simulink model "Bruening_4t_showshuffle"  (R2015a)
settings: Solver=ode4  SolverMode=MultiTasking  StartTime=0.0  StopTime=inf  FixedStep=BKIN_STEP_TIME  RelTol=1e-3
StartFcn:
  |  warndlg('Dexterit-E models cannot run under simulation. Please compile your model and run it from within Dexterit-E.');set_param(bdroot,'SimulationCommand','stop')
model workspace (MAT data in the model file):
  BKIN_STEP_TIME = 0.00025
  col_x = 1
  col_y = 2
  E_TARGET_ON = 3
  E_HOLD_AT_TARGET = 5
  LOGICAL_RADIUS = 4
  START_TARGET_COL = 1
  END_TARGET_COL = 2
  ROTATION_CENTER = 5
  WAIT_AT_1stTARGET_COL = 7
  MAXREACHTIME_COL = 8
  DELAY_POSTTRIAL_COL = 9
  E_STAY_CENTER = 2
  VISUAL_RADIUS = 3
  COLOR = 5
  ALTCOLOR = 6
  STROKECOLOUR = 7
  STROKEWIDTH = 9
  TARGET_EGG = 6
  LABEL_TEXT = 12
  LABEL_COLOUR = 13
  LABEL_HEIGHT = 14
  TEXT_DISPLAY_TARGET = 10
  ALTSTROKECOLOUR = 8
  SEGMENT_COUNT = 11
  E_TARGET_MISS = 6
  END_X = 10
  END_Y = 11
  E_LEFT_RING = 4
  E_START_BLOCK = 10
  BKIN_KINEMATIC_FRAME_SIZE = 400
  E_NO_EVENT = 1
  TARGET_IN_USE = 3
  R_PROB = 4
  E_R_TARG1 = 7
  E_M_TARG1 = 12
  E_R_TARG2 = 8
  E_M_TARG2 = 13
  E_R_TARG3 = 9
  E_M_TARG3 = 14
  E_R_TARG4 = 11
  E_M_TARG4 = 15
  WAIT_TIME = 12
  TONE_DURATION = 13
  FLASH_INTER = 14
  FLASH_NUM = 15
  BREAK_T1 = 16
  BREAK_T2 = 17
  ALTVISUAL_RADIUS = 15
  ALTCOLOR2 = 16
undefined symbols (not defined in the file or in its folder): slselsubs
libraries: Video x15, simulink x12, xpcrtudplib x12, xpcutilitieslib x10, xpcobsoletelib x8, ethercat x2, General x2, slrtlib x2, KINARM_general x1
(part 5 of 6)

== matlab function Bruening_4t_showshuffle/DataLogging/Poll KINARM/PMAC Subsystem/read_pmac/Robot_data_builder ==
  data: bR1HasSecondardy input; bR2HasSecondardy input; robot1Data input; robot2Data input; robot1PrimaryEncData input; robot2PrimaryEncData input; robot1DataOut output; robot2DataOut output; servoCounter input; plccVer input; robot1PrimaryEncDataOut output; robot2PrimaryEncDataOut output
function [robot1DataOut, robot2DataOut, robot1PrimaryEncDataOut, robot2PrimaryEncDataOut] = convertPMACValues(bR1HasSecondardy, bR2HasSecondardy, robot1Data, robot2Data, robot1PrimaryEncData, robot2PrimaryEncData, servoCounter, plccVer)

    persistent robot1Struct robot2Struct robot1StructPrimary robot2StructPrimary servoValuesR1 servoValuesR2
    
    if isempty(robot1Struct)
        robot1Struct = getStruct();
        robot2Struct = getStruct();
        robot1StructPrimary = getStruct();
        robot2StructPrimary = getStruct();
        servoValuesR1 = zeros(5, 1);
        servoValuesR2 = zeros(5, 1);
    end
    
    if plccVer < 7
        robot1DataOut = robot1Data;
        robot2DataOut = robot2Data;
        robot1PrimaryEncDataOut = robot1PrimaryEncData;
        robot2PrimaryEncDataOut = robot2PrimaryEncData;
        return
    end
    
    if servoCounter(1) ~= servoValuesR1(1)
        robot1Struct = updatePositions(robot1Struct, robot1Data, bR1HasSecondardy);
        robot1StructPrimary = updatePositions(robot1StructPrimary, robot1PrimaryEncData, 0);
        servoValuesR1 = insertVal(servoValuesR1, servoCounter(1));
        robot1Struct = calculateVelAcc(robot1Struct, servoValuesR1, robot1Data);
        robot1StructPrimary = calculateVelAcc(robot1StructPrimary, servoValuesR1, robot1PrimaryEncData);
    end
    
    if servoCounter(2) ~= servoValuesR2(1)
        robot2Struct = updatePositions(robot2Struct, robot2Data, bR2HasSecondardy);
        robot2StructPrimary = updatePositions(robot2StructPrimary, robot2PrimaryEncData, 0);
        servoValuesR2 = insertVal(servoValuesR2, servoCounter(2));
        robot2Struct = calculateVelAcc(robot2Struct, servoValuesR2, robot2Data);
        robot2StructPrimary = calculateVelAcc(robot2StructPrimary, servoValuesR2, robot2PrimaryEncData);
    end
    
    robot1DataOut = insertVelAcc(robot1Data, robot1Struct);
    robot2DataOut = insertVelAcc(robot2Data, robot2Struct);

    robot1PrimaryEncDataOut = insertVelAcc(robot1PrimaryEncData, robot1StructPrimary);
    robot2PrimaryEncDataOut = insertVelAcc(robot2PrimaryEncData, robot2StructPrimary);
    
    %We used to provide a filtered velocity, but we can't with EtherCAT and
    %it was not being used anywhere anyway. 
    robot1DataOut(7:8) = robot1DataOut(3:4);
    robot2DataOut(7:8) = robot2DataOut(3:4);
end


function robotDataOut = insertVelAcc(robotData, robotStruct)
    robotDataOut = robotData(:);
    robotDataOut(3) = robotStruct.shoVel(1);
    robotDataOut(4) = robotStruct.elbVel(1);
    robotDataOut(5) = robotStruct.shoAcc;
    robotDataOut(6) = robotStruct.elbAcc;
end

function st=getStruct()
    st = struct('shoPos', zeros(5, 1), 'elbPos', zeros(5, 1), ...
        'shoVel', zeros(5, 1), 'elbVel', zeros(5, 1), ...
        'shoAcc', 0, 'elbAcc', 0, 'bHasSecondary', 0);
end

function robotStruct = updatePositions(robotStruct, robotData, bHasSecondardy)
    robotStruct.shoPos = insertVal(robotStruct.shoPos, robotData(1));
    robotStruct.elbPos = insertVal(robotStruct.elbPos, robotData(2));
    robotStruct.bHasSecondary = bHasSecondardy;
end

function arr=insertVal(arr, v)
    arr = circshift(arr, 1);
    arr(1) = v;
end

function robotStructOut=calculateVelAcc(robotStruct, servoValues, robotData)
    %matches from PMAC code
    robotStructOut = robotStruct;
    servoTimeStep = (7427414.0/8388608.0) / 1000; 
    %do not name this anything that will make it the first variable name in
    %this method alphabetically. Seriously. With the name "duration" compiling
    %a model would work in 2010a, but nothing higher. Most models would compile,
    %but the verification task would not!
    stepDuration = 0;
    
    if robotStruct.bHasSecondary
        stepDuration = ((servoValues(1) - servoValues(2)) * servoTimeStep);
        if stepDuration == 0
            shoVel = robotStruct.shoVel(1);
            elbVel = robotStruct.elbVel(1);
        else
            shoVel = (robotStruct.shoPos(1) - robotStruct.shoPos(2)) / stepDuration;
            elbVel = (robotStruct.elbPos(1) - robotStruct.elbPos(2)) / stepDuration;        
        end
    else
        shoVel = robotData(3);
        elbVel = robotData(4);
    end
    
    robotStructOut.shoVel = insertVal(robotStruct.shoVel, shoVel);
    robotStructOut.elbVel = insertVal(robotStruct.elbVel, elbVel);

    if robotStruct.bHasSecondary        
        if stepDuration == 0
            shoAcc = robotStruct.shoAcc;
            elbAcc = robotStruct.elbAcc;
        else
            shoAcc = (robotStruct.shoVel(1) - robotStruct.shoVel(2)) / stepDuration;
            elbAcc = (robotStruct.elbVel(1) - robotStruct.elbVel(2)) / stepDuration;        
        end
    else
        stepDuration = ((servoValues(1) - servoValues(5)) * servoTimeStep);
        shoAcc = (robotStruct.shoVel(1) - robotStruct.shoVel(5)) / stepDuration;
        elbAcc = (robotStruct.elbVel(1) - robotStruct.elbVel(5)) / stepDuration;        
    end    
    
    robotStructOut.shoAcc = shoAcc;
    robotStructOut.elbAcc = elbAcc;
end

== matlab function Bruening_4t_showshuffle/DataLogging/Poll KINARM/PMAC Subsystem/read_pmac/filter_velocities ==
  data: robot1Data input; robot2Data input; robot1DataOut output; robot2DataOut output; servoCounters input; plccVer input
function [robot1DataOut, robot2DataOut] = filterVelocities(robot1Data, robot2Data, servoCounters, plccVer)

    persistent robot1Struct robot2Struct
    POLES = 2;
    
    if isempty(robot1Struct)
        robot1Struct = getStruct(POLES);
        robot2Struct = getStruct(POLES);
    end
    
    if plccVer < 7
        robot1DataOut = robot1Data;
        robot2DataOut = robot2Data;
        return
    end
    
    robot1DataOut = robot1Data(:);
    robot2DataOut = robot2Data(:);
    
    robot1Struct = updateValues(robot1Struct, robot1Data, servoCounters(1), POLES);
    robot2Struct = updateValues(robot2Struct, robot2Data, servoCounters(2), POLES);
        
    %We used to provide a filtered velocity, but we can't with EtherCAT and
    %it was not being used anywhere anyway. 
    robot1DataOut(7:8) = [robot1Struct.shoVelFilt(POLES + 1), robot1Struct.elbVelFilt(POLES + 1)];
    robot2DataOut(7:8) = [robot2Struct.shoVelFilt(POLES + 1), robot2Struct.elbVelFilt(POLES + 1)];
end


function st=getStruct(poles)
    valueCount = poles + 1;
    st = struct('shoVel', zeros(valueCount, 1), 'elbVel', zeros(valueCount, 1), ...
        'shoVelFilt', zeros(valueCount, 1), 'elbVelFilt', zeros(valueCount, 1), ...
        'servoCounter', zeros(valueCount, 1));
end

function arr=insertVal(arr, v)
    arr = circshift(arr, -1);
    arr(length(arr)) = v;
end

function robotStruct = updateValues(robotStruct, robotData, servoCounter, POLES)
    if servoCounter == robotStruct.servoCounter(POLES + 1)
        return
    end
    
    robotStruct.servoCounter = insertVal(robotStruct.servoCounter, servoCounter);
    
    [robotStruct.shoVel, robotStruct.shoVelFilt] = filterJoint(robotStruct.shoVel, robotStruct.shoVelFilt, robotData(3), POLES);
    [robotStruct.elbVel, robotStruct.elbVelFilt] = filterJoint(robotStruct.elbVel, robotStruct.elbVelFilt, robotData(4), POLES);
end

function [velocitiesOut, velFilt] = filterJoint(velocities, filtVelocities, newVelocity, POLES)

%all filter constants from http://www-users.cs.york.ac.uk/~fisher/cgi-bin/mkfscript

    %GAIN = 4.143204922e+03; % 1KHz gain
    GAIN = 1.342624471e+03; %1.129 KHz gain (PMAC speed)
    
    %FILTER_VALUES = [-0.9565436765, 1.9555782403]; % 1KHz
    FILTER_VALUES = [-0.9243128082, 1.9213335686]; % 1.129 KHz
    
    velocitiesOut = insertVal(velocities, newVelocity / GAIN);
    velFilt = insertVal(filtVelocities, 0);

    velFilt(POLES + 1) = velocitiesOut(1) + ...
         velocitiesOut(2) * 2.0 + ...
         velocitiesOut(3) + ...
         velFilt(1) * FILTER_VALUES(1) + ...
         velFilt(2) * FILTER_VALUES(2);
    
     if isnan(velFilt(POLES + 1)) || isinf(velFilt(POLES + 1))
         velFilt(POLES + 1) = 0;
    end
end

== matlab function Bruening_4t_showshuffle/DataLogging/Poll KINARM/PMAC Subsystem/update settings/update status format ==
  data: pmacStatus input; outStatus output
function outStatus = fcn(pmacStatus)
%#eml

outStatus = zeros(1, 7, 'uint32');
outStatus(5:6) = pmacStatus(2:3);

STATUS_FUNCTIONING = uint32(0);
STATUS_READY = uint32(1);
STATUS_FAULTED = uint32(2);

%Each motor has 2 possible states: 0 working, 1 faulted. The READY state is only used by EtherCAT
for n=0:3
    motor = bitand( bitshift(pmacStatus(1), -n), 1);
    if motor == 1
       outStatus(n + 1) =  STATUS_FAULTED;
    else
        outStatus(n + 1) = STATUS_FUNCTIONING;
    end
end

== matlab function Bruening_4t_showshuffle/DataLogging/Poll KINARM/constants/arm1/decode robot ==
  data: system_type input; robot_type input; isEP output; robot_version input; isHumanEXO output; isNHPEXO output; isClassicExo output; isUTSEXO output; isPMAC output; isECAT output
function [isEP, isHumanEXO, isNHPEXO, isClassicExo, isUTSEXO, isPMAC, isECAT] = fcn(system_type, robot_type, robot_version)
%#eml
isEP = 0;
isHumanEXO = 0;
isNHPEXO = 0;
isClassicExo = 0;
isUTSEXO = 0;
isPMAC = 0;
isECAT = 0;

if robot_type == 0
    isHumanEXO = 1;    
    if robot_version == 1
        isClassicExo = 1;        
    elseif robot_version == 2
        isUTSEXO = 1;
    end    
elseif robot_type == 1
    isEP = 1;
elseif robot_type == 2
    isNHPEXO = 1;        
    if robot_version == 1
        isClassicExo = 1;        
    elseif robot_version == 2
        isUTSEXO = 1;
    end
end

if system_type == 1
   isPMAC = 1;
elseif system_type == 2
    isECAT = 1;
end

== matlab function Bruening_4t_showshuffle/DataLogging/Poll KINARM/constants/arm2/decode robot ==
  data: system_type input; robot_type input; isEP output; robot_version input; isHumanEXO output; isNHPEXO output; isClassicExo output; isUTSEXO output; isPMAC output; isECAT output
function [isEP, isHumanEXO, isNHPEXO, isClassicExo, isUTSEXO, isPMAC, isECAT] = fcn(system_type, robot_type, robot_version)
%#eml
isEP = 0;
isHumanEXO = 0;
isNHPEXO = 0;
isClassicExo = 0;
isUTSEXO = 0;
isPMAC = 0;
isECAT = 0;

if robot_type == 0
    isHumanEXO = 1;    
    if robot_version == 1
        isClassicExo = 1;        
    elseif robot_version == 2
        isUTSEXO = 1;
    end    
elseif robot_type == 1
    isEP = 1;
elseif robot_type == 2
    isNHPEXO = 1;        
    if robot_version == 1
        isClassicExo = 1;        
    elseif robot_version == 2
        isUTSEXO = 1;
    end
end

if system_type == 1
   isPMAC = 1;
elseif system_type == 2
    isECAT = 1;
end

== matlab function Bruening_4t_showshuffle/DataLogging/Poll Force Plates/plate2/parse packet 1 ==
  data: packet input; forces output; moments output; timer output; calibration input; gain input; ain_slope input; ain_offset input; orientation input; zero_voltage input
function [forces, moments, timer] = fcn(packet, calibration, gain, ain_slope, ain_offset, orientation, zero_voltage)
    %This pulls voltages and timer infomation from the packet we got back from
    %the lab jack.
    
    voltages = zeros(1, 8);
    timers = zeros(1, 3);

    for n = 1:8
        bits = readUShort(packet, 13 + ((n - 1)*2));
        voltages(n) = binaryToCalibratedAnalogVoltage(bits, ain_slope, ain_offset);
    end
    
    for n = 1:3
        timers(n) = readUInt(packet, 53 + ((n - 1)*4));
    end
    
    %convert the time stamp to a time in seconds.
    timer = timers(1) / 750000.0; 
    
    %all voltages are between -2.5 to 2.5, here we are normalizeing what we read to zero.
    voltages = voltages - zero_voltage;
    voltages = voltages(1:8); % only the first 8 channels matter.
    
    %using the calibration matrix we convert the to the forces and moments
    values = calibration * (voltages / gain)';
    forces = values(1:3);
    moments = values(4:6);
    
	%reverse the Z force to get it into global coordinates.
	forces(3) = -forces(3);

	%considering the positions of the cables push all measures into global coordinates
    if orientation == 0
        forces(2) = -forces(2);
        moments(2) = -moments(2);
    elseif orientation == 90
        y = forces(2);
        forces(2) = -forces(1);
        forces(1) = -y;

        y = moments(2);
        moments(2) = -moments(1);
        moments(1) = -y;
	elseif orientation == 180
        forces(1) = -forces(1);        
        moments(1) = -moments(1);        
    elseif orientation == 270
        y = forces(2);
        forces(2) = forces(1);
        forces(1) = y;

		y = moments(2);
        moments(2) = moments(1);
        moments(1) = y;
    end
end

function val = readUShort(data, offset)
    p1 = uint32(data(offset));
    p2 = uint32(data(offset + 1));
    val = double(p1 + (p2 * 256));
end

function val = readUInt(data, offset)
    p1 = uint32(data(offset));
    p2 = uint32(data(offset + 1));
    p3 = uint32(data(offset + 2));
    p4 = uint32(data(offset + 3));
    val = double(p1 + (p2 * 256) + (p3 * 2^16) + (p4 * 2^24));
end

function voltage = binaryToCalibratedAnalogVoltage(bits, ain_slope, ain_offset)
    voltage = (bits * ain_slope) + ain_offset;
end

== matlab function Bruening_4t_showshuffle/DataLogging/Poll KINARM/createKINData/Create KINARM Data Array ==
  data: robot_calibrations input; robot_hardware_settings input; force_sensor_data input; robot_data input; servo_update_count input; delay_estimates input; primary_encoder_data input; ep_calibration_button_bitfield input; torque_command input; hand_feedback_settings input; kinarm_data output; dominant_arm input; primary_encoder_data_out output; gaze_data input
% This function constructs a matrix of KINARM-related data called "KINdata". This matrix consists of three rows: the first two are each
% for data related to the respective robot (i.e. row 1 is for robot 1 data, row 2 for robot 2 data, etc.), and the third row is for data
% not specific to either arm. Each row of the matrix is currently of length 50, though not all elements in each row are used.
function [kinarm_data, primary_encoder_data_out]= create_KINARM_data_array(robot_calibrations, robot_hardware_settings, force_sensor_data, ...
                                                      robot_data, servo_update_count, delay_estimates, primary_encoder_data, ...
                                                      ep_calibration_button_bitfield, torque_command, hand_feedback_settings, dominant_arm, gaze_data)

kinarm_data = zeros(3,50);
primary_encoder_data_out = zeros(2,6);

% Create the rows of robot-specific data. The utility function create_robot_row is used to assemble the values for each row. 
% The last section of that function (in which the row elements are assigned individually) documents the row contents.
kinarm_data(1,:) = create_robot_row(robot_calibrations(1:8), robot_hardware_settings(1:12), ...
                                    force_sensor_data(1:7), robot_data(1:10), torque_command(1:2));

kinarm_data(2,:) = create_robot_row(robot_calibrations(9:16), robot_hardware_settings(13:24), ...
                                    force_sensor_data(8:14), robot_data(11:20), torque_command(3:4));
								
% Create the last row of KINdata, which contains information not specific to any single arm.
kinarm_data(3,1) = dominant_arm;                     % dominant KINARM for the experiment (1: arm 1, 2: arm 2)
kinarm_data(3,2) = hand_feedback_settings(5);        % duration of feed forward for position of hand feedback (s)
kinarm_data(3,3) = hand_feedback_settings(1);        % hand feedback arm (0: none, 1: dominant, 2: non-dominant, 3: both, 4: controlled by task program)
kinarm_data(3,4) = hand_feedback_settings(2);        % hand feedback settings source (0: GUI, 1: from task program)
kinarm_data(3,5) = hand_feedback_settings(4);        % feedback colour (RRRGGGBBB string converted to integer)
kinarm_data(3,6) = hand_feedback_settings(3);        % feedback radius (m)
kinarm_data(3,7) = 1;                                % global load enable set by BKIN client software (no longer an option; thus always on)
kinarm_data(3,8) = delay_estimates(1);               % primary encoders velocity delay estimate (s)
kinarm_data(3,9) = delay_estimates(2);               % primary encoders acceleration delay estimate (s)
kinarm_data(3,10) = delay_estimates(3);              % secondary encoders velocity delay estimate (s)
kinarm_data(3,11) = delay_estimates(4);              % secondary encoders acceleration delay estimate (s)
kinarm_data(3,12) = servo_update_count;              % servo update count
kinarm_data(3,13) = ep_calibration_button_bitfield;  % EP calibration button status bitfield

gaze_available = gaze_data(1);
kinarm_data(3,14) = gaze_available;              % is Gaze tracking hardware available
kinarm_data(3,15) = hand_feedback_settings(6);   % Gaze feedback (0: on, 1: controlled by task program)

if gaze_available
    kinarm_data(3,16) = gaze_data(2);            % Gaze X location in global coordinates
    kinarm_data(3,17) = gaze_data(3);            % Gaze Y location in global coordinates
    kinarm_data(3,18) = gaze_data(4);            % Gaze Timestamp in seconds
    kinarm_data(3,19) = gaze_data(5);            % Gaze pupil area
    kinarm_data(3,20) = gaze_data(6);          % Gaze Event ID
    kinarm_data(3,21) = gaze_data(7);          % Gaze Event start time in seconds
    kinarm_data(3,22) = gaze_data(8);          % Gaze Event end time in seconds    
else
    kinarm_data(3,16) = -100;                    % Gaze X location in global coordinates
    kinarm_data(3,17) = -100;                    % Gaze Y location in global coordinates
    kinarm_data(3,18) = -100;                    % Gaze Timestamp in seconds
    kinarm_data(3,19) = -100;                    % Gaze Timestamp in seconds
end

% Create the two rows of primary encoder data. These outputs are analogous to the L1/L2 outputs in kinarm_data, the difference being that
% these are always derived from the primary encoders while the contents of kinarm_data is derived from the primary or secondary encoders
% (depending on the user's choice of whether or not to use the secondary encoders in the GUI).
for i = 1:2
	offset = (i-1)*6;
    
    relative_shoulder_angle = primary_encoder_data(1 + offset);
    relative_elbow_angle = primary_encoder_data(2 + offset);
    shoulder_velocity = primary_encoder_data(3 + offset);
    elbow_velocity = primary_encoder_data(4 + offset);
    shoulder_acceleration = primary_encoder_data(5 + offset);
    elbow_acceleration = primary_encoder_data(6 + offset);

    shoulder_angle_offset = robot_calibrations(1 + (i-1)*8);
    elbow_angle_offset = robot_calibrations(2 + (i-1)*8);
	L1 = robot_calibrations(5 + (i-1)*8);                               % L1 (upper arm segment) length (m)
	L3_error = robot_calibrations(8 + (i-1)*8);                         % L3 error, the difference between lengths L3 and L5 (m)
    
    hwoffset = (i-1)*12;
	robot_orientation = robot_hardware_settings(6 + hwoffset);          % robot orientation (1: right-handed from robot perspective, -1: left-handed from robot perspective)
 	L5 = robot_hardware_settings(3 + hwoffset);                         % L5 segment length (m)
	L2_L5_angle = robot_hardware_settings(4 + hwoffset);                % angle of L2 relative to L5 (rad)
    robot_type = robot_hardware_settings(1 + hwoffset);
    isExo = robot_type == 0 || robot_type == 2;
    
	% Before proceeding, the shoulder and elbow angles are shifted by the offsets determined by the calibration. If the calibration has been
	% performed correctly, this ensures that the angle of 0 corresponds to when the arm is aligned with the coronal plane. In the case of the 
	% elbow angle for a KINARM EXO, an extra correction is performed (using a utility function, and according to the current calibration) to 
	% account for small imperfections in the parallelogram of KINARM links caused by differences in the lengths of L3 and L5 (which are 
	% theoretically equal).
	shoulder_angle = relative_shoulder_angle + shoulder_angle_offset;

	% If the robot is an Exoskeleton, use the correct_elbow_angle function to account for imperfections on the KINARM robot parallelogram structure
	if isExo  
		[angle_corr, vel_corr, acc_corr] = correct_elbow_angle(relative_elbow_angle + elbow_angle_offset, elbow_velocity, elbow_acceleration, L2_L5_angle, L1, L5, L3_error);				
		elbow_angle = relative_elbow_angle + elbow_angle_offset + angle_corr;
		elbow_velocity = elbow_velocity + vel_corr;
		elbow_acceleration = elbow_acceleration + acc_corr;		
	else
		elbow_angle = relative_elbow_angle + elbow_angle_offset;
	end

    L1_angle = shoulder_angle;
    L2_angle = shoulder_angle + elbow_angle;

    L1_velocity = shoulder_velocity;
    L2_velocity = shoulder_velocity + elbow_velocity;

    L1_acceleration = shoulder_acceleration;
    L2_acceleration = shoulder_acceleration + elbow_acceleration;

	% a robot_orientation < 0 means that the robot is left-handed from its perspective (i.e. if you look at the robot structure, 
	% and pretend that it is a humanoid, the robot itself looks left-handed).  For an Exoskeleton robot, this is the
	% robot that the left-hand of the subject grabs. For an EP robot, this is the robot that the subjec'ts right-hand grabs.  
	
    if robot_orientation < 0
        L1_angle = -L1_angle + pi;
        L2_angle = -L2_angle + pi;

        L1_velocity = -L1_velocity;
        L2_velocity = -L2_velocity;

        L1_acceleration = -L1_acceleration;
        L2_acceleration = -L2_acceleration;
    end

    primary_encoder_data_out(i,1) = L1_angle;
    primary_encoder_data_out(i,2) = L2_angle;
    
    primary_encoder_data_out(i,3) = L1_velocity;
    primary_encoder_data_out(i,4) = L2_velocity;
    
    primary_encoder_data_out(i,5) = L1_acceleration;
    primary_encoder_data_out(i,6) = L2_acceleration;
end


%%%%%%%%%%%%%%%%%%%%%%%%%%%%%%%%%%%%%%%%%%%%%%%%%%%%%%%%%%%%%%%%%%%%%%%%%%%%%%%%%%%%%%%%%%%%%%%%%%%%%%%%%%%%%%%%%%%%%%%%
%%%%%%%%%%%%%%%%%%%%%%%%%%%%%%%%%%%%%%%%%%%%%%%%%%%%%%%%%%%%%%%%%%%%%%%%%%%%%%%%%%%%%%%%%%%%%%%%%%%%%%%%%%%%%%%%%%%%%%%%
% This function creates a row of arm-specific data for the KINARM data matrix. 
function robot_row = create_robot_row(calibration, hardware_settings, force_sensor_data, robot_data, torque_command)

% Extract the relevant information from each input array.
shoulder_angle_offset = calibration(1);            % offset added to motion control card shoulder angle to get real angle (rad)
elbow_angle_offset = calibration(2);               % offset added to motion control card elbow angle to get real angle (rad)
shoulder_position_x = calibration(3);              % shoulder x position (m) (global coordinates)
shoulder_position_y = calibration(4);              % shoulder y position (m) (global coordinates)
L1 = calibration(5);                               % L1 (upper arm segment) length (m)
L2 = calibration(6);                               % L2 (forearm segment) length (m); segment length puts distal end in line with subject pointer
pointer_offset = calibration(7);                   % perpendicular distance from L2 to subject pointer (m)
L3_error = calibration(8);                         % L3 error, the difference between lengths L3 and L5 (m)

robot_type = hardware_settings(1);                 % robot type (0: EXO, 1: EP, 2:NHP)
isExo = robot_type == 0 || robot_type == 2;
isEP = robot_type == 1;
L5 = hardware_settings(3);                         % L5 segment length (m)
L2_L5_angle = hardware_settings(4);                % angle of L2 relative to L5 (rad)
force_sensor_angle_offset = hardware_settings(5);  % offset of force sensor from forearm linkage (rad)
robot_orientation = hardware_settings(6);          % robot orientation (1: right-handed from robot perspective, -1: left-handed from robot perspective)

force_sensor_force_u = force_sensor_data(1);       % force sensor u force (N)
force_sensor_force_v = force_sensor_data(2);       % force sensor v force (N)
force_sensor_force_w = force_sensor_data(3);       % force sensor w force (N)
force_sensor_torque_u = force_sensor_data(4);      % force sensor u torque (Nm) 
force_sensor_torque_v = force_sensor_data(5);      % force sensor v torque (Nm)
force_sensor_torque_w = force_sensor_data(6);      % force sensor w torque (Nm)
force_sensor_timestamp = force_sensor_data(7);      % force sensor w torque (Nm)

relative_shoulder_angle = robot_data(1);        % current shoulder joint angle (rad)
relative_elbow_angle = robot_data(2);           % current elbow joint angle (rad)
shoulder_velocity = robot_data(3);                 % shoulder joint angular velocity (rad/s)
elbow_velocity = robot_data(4);                    % elbow joint angular velocity (rad/s)
shoulder_acceleration = robot_data(5);             % shoulder joint angular acceleration (rad/s^2)
elbow_acceleration = robot_data(6);                % elbow joint angular acceleration (rad/s^2)
filtered_shoulder_velocity = robot_data(7);        % filtered shoulder velocity (rad/s)
filtered_elbow_velocity = robot_data(8);           % filtered elbow velocity (rad/s)
motor1_status = robot_data(9);                     % motor 1 status
motor2_status = robot_data(10);                    % motor 2 status

shoulder_torque_cmd = torque_command(1);	       % commanded shoulder torque (Nm)
elbow_torque_cmd = torque_command(2);              % commanded elbow torque (Nm)



% With the inputs unpacked, start using them to compute other values that will be included in the data array. Some inputs are included in the
% array directly, but the kinematic data is also developed from the joint-based information supplied by the polling function into information 
% about the arm segments, the elbow, and the hand/fingertip as described in the following sections.

% Before proceeding, the shoulder and elbow angles are shifted by the offsets determined by the calibration. If the calibration has been
% performed correctly, this ensures that the angle of 0 corresponds to when the arm is aligned with the coronal plane. In the case of the 
% elbow angle for a KINARM EXO, an extra correction is performed (using a utility function, and according to the current calibration) to 
% account for small imperfections in the parallelogram of KINARM links caused by differences in the lengths of L3 and L5 (which are 
% theoretically equal).
shoulder_angle = relative_shoulder_angle + shoulder_angle_offset;

% If the robot is an Exoskeleton, use the correct_elbow_angle function to account for imperfections on the KINARM robot parallelogram structure
if isExo
	[angle_corr, vel_corr, acc_corr] = correct_elbow_angle(relative_elbow_angle + elbow_angle_offset, elbow_velocity, elbow_acceleration, L2_L5_angle, L1, L5, L3_error);
	elbow_angle = relative_elbow_angle + elbow_angle_offset + angle_corr;
	elbow_velocity = elbow_velocity + vel_corr;
	elbow_acceleration = elbow_acceleration + acc_corr;
else
	elbow_angle = relative_elbow_angle + elbow_angle_offset;
end

% Convert robot orientation as supplied in the hardware settings (a scaling factor used to calculate robot data) to the number 1 or 2,
% indicating which of the subject's arms will normally be using the robot: right or left, respectively. This is done to be consistent 
% with previous versions of the TDK. Note that the robot orientations of KINARM EP robots are "opposite" those for KINARM EXOs when.
if (isEP && robot_orientation < 0.0) || (isExo && robot_orientation > 0.0)
    arm_orientation = 1;  % right arm orientation expected for subject
else
    arm_orientation = 2;  % left arm orientation expected for subject
end

% Create a motor status variable for the robot that is consistent with previous versions of the TDK: the value forms a bitfield in
% which non-zero bits indicate a motor is disabled or faulted. The least significant bit is motor 1; the next is motor 2.
motor_status = motor2_status * 2 + motor1_status;

% Calculate segment information, i.e. positions, velocities, and accelerations for L1 and L2. "Segment-based" values here differ from the
% "joint-based" values in a few ways, though they are still expressed in angles:
%   i) elbow angles are no longer shoulder-relative (that is, L2 angles are not relative to L1)
%  ii) positions are expressed with the corrections calculated above
% iii) all angles are expressed in the same system, where 0 is the angular position of the exoskeleton right arm when aligned with the 
%      coronal plane and positive changes in angle correspond to counterclockwise movements.
%
% This section also determines the torque commands for motor 1 (shoulder) and motor 2 (elbow). When a positive torque is applied to the 
% forearm linkage by motor 2 it causes the same positive force on the upper arm linkage, so the torque applied to motor 1 is the desired
% shoulder torque less any torque commanded at the elbow.

L1_angle = shoulder_angle;
L2_angle = shoulder_angle + elbow_angle;

pointer_angle = shoulder_angle + elbow_angle + pi/2;
    
L1_velocity = shoulder_velocity;
L2_velocity = shoulder_velocity + elbow_velocity;
	
L1_acceleration = shoulder_acceleration;
L2_acceleration = shoulder_acceleration + elbow_acceleration;
    
M1_torque_cmd = shoulder_torque_cmd - elbow_torque_cmd;
M2_torque_cmd = elbow_torque_cmd;

% a robot_orientation < 0 means that the robot is left-handed from its perspective (i.e. if you look at the robot structure, 
% and pretend that it is a humanoid, the robot itself looks left-handed).  For an Exoskeleton robot, this is the
% robot that the left-hand of the subject grabs. For an EP robot, this is the robot that the subjec'ts right-hand grabs.  

if (robot_orientation == -1)
    L1_angle = -L1_angle + pi;
    L2_angle = -L2_angle + pi;
    
    pointer_angle = -pointer_angle + pi;
    
    L1_velocity = -L1_velocity;
    L2_velocity = -L2_velocity;
    
    L1_acceleration = -L1_acceleration;
    L2_acceleration = -L2_acceleration;
    
    M1_torque_cmd = -M1_torque_cmd;
    M2_torque_cmd = -M2_torque_cmd;
end

% Calculate elbow information, i.e. position, velocity, and acceleration, in X-Y space rather than joint angles.
elbow_position_x = shoulder_position_x + (L1 * cos(L1_angle));
elbow_position_y = shoulder_position_y + (L1 * sin(L1_angle));

elbow_velocity_x = -L1 * sin(L1_angle) * L1_velocity;
elbow_velocity_y =  L1 * cos(L1_angle) * L1_velocity;

elbow_acceleration_x = -L1 * (( cos(L1_angle) * L1_velocity^2) + (sin(L1_angle) * L1_acceleration));
elbow_acceleration_y =  L1 * ((-sin(L1_angle) * L1_velocity^2) + (cos(L1_angle) * L1_acceleration));

% Calculate fingertip/subject pointer/hand feedback information, i.e. position, velocity, and acceleration, in X-Y space.
hand_position_x = elbow_position_x + (L2 * cos(L2_angle)) + (pointer_offset * cos(pointer_angle));
hand_position_y = elbow_position_y + (L2 * sin(L2_angle)) + (pointer_offset * sin(pointer_angle));

hand_velocity_x = elbow_velocity_x - (L2 * sin(L2_angle) * L2_velocity) - (pointer_offset * sin(pointer_angle) * L2_velocity);
hand_velocity_y = elbow_velocity_y + (L2 * cos(L2_angle) * L2_velocity) + (pointer_offset * cos(pointer_angle) * L2_velocity);

hand_acceleration_x = elbow_acceleration_x - (L2 * (( cos(L2_angle) * L2_velocity^2) + (sin(L2_angle) * L2_acceleration))) - ...
    (pointer_offset * (( cos(pointer_angle) * L2_velocity^2) + (sin(pointer_angle) * L2_acceleration)));
hand_acceleration_y = elbow_acceleration_y + (L2 * ((-sin(L2_angle) * L2_velocity^2) + (cos(L2_angle) * L2_acceleration))) + ...
    (pointer_offset * ((-sin(pointer_angle) * L2_velocity^2) + (cos(pointer_angle) * L2_acceleration)));

% Calculate force sensor data for EP robots, or zero it for EXO robots. On each EP robot the force sensor is mounted at known angle to 
% the forearm linkage, which is specified as an input to this block. Two variants of the data are calculated: i) scaled in the force 
% sensor's local coordinate system ("uvw"), and ii) transformed to be in the global coordinate system ("xyz").
if isEP
    
    force_sensor_force_u = force_sensor_force_u / 1000000.0;  % scale values to SI using factors defined in force sensor configurations
    force_sensor_force_v = force_sensor_force_v / 1000000.0;
    force_sensor_force_w = force_sensor_force_w / 1000000.0;

    force_sensor_torque_u = force_sensor_torque_u / 1000000.0;
    force_sensor_torque_v = force_sensor_torque_v / 1000000.0;
    force_sensor_torque_w = force_sensor_torque_w / 1000000.0;

    sensor_u_angle = L2_angle - force_sensor_angle_offset;
    sensor_v_angle = L2_angle - force_sensor_angle_offset - pi/2;
    
    force_sensor_force_x = force_sensor_force_u * cos(sensor_u_angle) + force_sensor_force_v * cos(sensor_v_angle);
    force_sensor_force_y = force_sensor_force_u * sin(sensor_u_angle) + force_sensor_force_v * sin(sensor_v_angle);
    force_sensor_force_z = -force_sensor_force_w;

    force_sensor_torque_x = double(force_sensor_torque_u * cos(sensor_u_angle) + force_sensor_torque_v * cos(sensor_v_angle));
    force_sensor_torque_y = double(force_sensor_torque_u * sin(sensor_u_angle) + force_sensor_torque_v * sin(sensor_v_angle));
    force_sensor_torque_z = double(-force_sensor_torque_w);
    
else
    force_sensor_force_u = 0.0;
    force_sensor_force_v = 0.0;
    force_sensor_force_w = 0.0;

    force_sensor_torque_u = 0.0;
    force_sensor_torque_v = 0.0;
    force_sensor_torque_w = 0.0;

    force_sensor_force_x = 0.0;
    force_sensor_force_y = 0.0;
    force_sensor_force_z = 0.0;

    force_sensor_torque_x = 0.0;
    force_sensor_torque_y = 0.0;
    force_sensor_torque_z = 0.0;
end

% Construct the arm data array. Its construction is laid out here explicitly to provide comments for each entry (some are repeats from above). 
robot_row = zeros(1,50);

robot_row(1,1) = L1;                            % L1 (upper arm segment) length (m)
robot_row(1,2) = L2;                            % L2 (forearm segment) length (m); segment length puts distal end in line with subject pointer
robot_row(1,3) = pointer_offset;                % perpendicular distance from L2 to subject pointer (m)
robot_row(1,4) = shoulder_position_x;           % shoulder x position (m) (global coordinates)
robot_row(1,5) = shoulder_position_y;           % shoulder y position (m) (global coordinates)
robot_row(1,6) = arm_orientation;               % subject's expected arm orientation (1: right, 2: left)
robot_row(1,7) = shoulder_angle;				% shoulder joint angle, with correction for offsets (see above) (rad)
robot_row(1,8) = elbow_angle;					% elbow joint angle, with correction for offsets (see above) (rad)
robot_row(1,9) = shoulder_velocity;             % shoulder joint angular velocity (rad/s)
robot_row(1,10) = elbow_velocity;               % elbow joint angular velocity (rad/s)
robot_row(1,11) = shoulder_acceleration;        % shoulder joint angular acceleration (rad/s^2)
robot_row(1,12) = elbow_acceleration;           % elbow joint angular acceleration (rad/s^2)
robot_row(1,13) = shoulder_torque_cmd;          % commanded shoulder torque (Nm)
robot_row(1,14) = elbow_torque_cmd;             % commanded elbow torque (Nm)
robot_row(1,15) = M1_torque_cmd;                % commanded motor 1 torque (shoulder torque less elbow torque) (Nm)
robot_row(1,16) = M2_torque_cmd;                % commanded motor 2 torque (Nm)
robot_row(1,17) = L1_angle;                     % upper arm angle with corrections, orientation-independent (see above) (rad)
robot_row(1,18) = L2_angle;                     % forearm angle with corrections, orientation and shoulder-independent (see above) (rad)
robot_row(1,19) = L1_velocity;                  % upper arm angular velocity, orientation-independent (see above) (rad/s)
robot_row(1,20) = L2_velocity;                  % forearm angular velocity, orientation and shoulder-independent (see above) (rad/s)
robot_row(1,21) = L1_acceleration;              % upper arm angular acceleration, orientation-independent (see above) (rad/s^2)
robot_row(1,22) = L2_acceleration;              % forearm angular acceleration, orientation and shoulder-independent (see above) (rad/s^2)
robot_row(1,23) = hand_position_x;              % fingertip position in x (m)
robot_row(1,24) = hand_position_y;              % fingertip position in y (m)
robot_row(1,25) = hand_velocity_x;              % fingertip velocity in x (m/s)
robot_row(1,26) = hand_velocity_y;              % fingertip velocity in y (m/s)
robot_row(1,27) = hand_acceleration_x;          % fingertip acceleration in x (m/s^2)
robot_row(1,28) = hand_acceleration_y;          % fingertip acceleration in y (m/s^2)
robot_row(1,29) = elbow_position_x;             % elbow position in x (m)
robot_row(1,30) = elbow_position_y;             % elbow position in y (m)
robot_row(1,31) = elbow_velocity_x;             % elbow velocity in x (m/s)
robot_row(1,32) = elbow_velocity_y;             % elbow velocity in y (m/s)
robot_row(1,33) = elbow_acceleration_x;         % elbow acceleration in x (m/s^2)
robot_row(1,34) = elbow_acceleration_y;         % elbow acceleration in y (m/s^2)
robot_row(1,35) = filtered_shoulder_velocity;   % filtered shoulder velocity from motion control card (rad/s)
robot_row(1,36) = filtered_elbow_velocity;      % filtered elbow velocity from motion control card (rad/s)
robot_row(1,37) = motor_status;                 % motor status (bitfield; each 0: motor enabled, 1: motor disabled/faulted)
robot_row(1,38) = force_sensor_force_u;         % force measured by force sensor along u in its local coordinate system (N)
robot_row(1,39) = force_sensor_force_v;         % force measured by force sensor along v in its local coordinate system (N)
robot_row(1,40) = force_sensor_force_w;         % force measured by force sensor along w in its local coordinate system (N)
robot_row(1,41) = force_sensor_torque_u;        % torque measured by force sensor along u in its local coordinate system (Nm)
robot_row(1,42) = force_sensor_torque_v;        % torque measured by force sensor along v in its local coordinate system (Nm)
robot_row(1,43) = force_sensor_torque_w;        % torque measured by force sensor along w in its local coordinate system (Nm)
robot_row(1,44) = force_sensor_force_x;         % force measured by force sensor along x in the global coordinate system (N)
robot_row(1,45) = force_sensor_force_y;         % force measured by force sensor along y in its local coordinate system (N)
robot_row(1,46) = force_sensor_force_z;         % force measured by force sensor along z in its local coordinate system (N)
robot_row(1,47) = force_sensor_torque_x;        % torque measured by force sensor along x in its local coordinate system (Nm)
robot_row(1,48) = force_sensor_torque_y;        % torque measured by force sensor along y in its local coordinate system (Nm)
robot_row(1,49) = force_sensor_torque_z;        % torque measured by force sensor along z in its local coordinate system (Nm)
robot_row(1,50) = force_sensor_timestamp;       % The timestamp from the force sensor(s)



function [angle_corr vel_corr acc_corr] = correct_elbow_angle(elbow_angle, elbow_vel, elbow_acc, theta2_5, L1, L5, L3_error)

% this function corrects for errors in non-perfect parallelogram structure
% It assumes that L5 is exact (because it is machined from one
% piece of material) and that there is an error in L3.  Note: although
% there could also be an error in L4, this 'correction' factor can
% effectively account for both errors by computing an equivalent L3_error

L3 = L5 + L3_error;

theta1_3 = theta2_5 - elbow_angle;		%actual angle between links 1 and 3
dtheta1_3dt = - elbow_vel;
d2theta1_3d2t = - elbow_acc;

% The following shifts theta1_3 to between -pi and pi and stores the shift.
% Although theta1_3 should always be between 0 and pi, during initial
% calibration there might be some values outside of that range.
theta1_3_2pi_offset = floor( (theta1_3 + pi)/(2 *pi) );
theta1_3 = theta1_3 - theta1_3_2pi_offset * 2 * pi;

%Option 1a
a = 4 * L3 * L5 - 4*L1*L5*cos(theta1_3);
b = -4 * L1 * L5 * sin(theta1_3);
c = L3^2 + L5^2 - 2 * L3 * L5 - 2 * L1 * L3_error * cos(theta1_3) ;

dbdt = -4 * L1 * L5 * cos(theta1_3) * dtheta1_3dt;
dcdt = 2 * L1 * L3_error * sin(theta1_3) * dtheta1_3dt;

d2bdt2 = 4 * L1 * L5 * sin(theta1_3) * dtheta1_3dt^2 -4 * L1 * L5 * cos(theta1_3) * d2theta1_3d2t;
d2cdt2 = 2 * L1 * L3_error * cos(theta1_3) * dtheta1_3dt^2 + 2 * L1 * L3_error * sin(theta1_3) * d2theta1_3d2t;

sqroot = sqrt( b^2 - 4 * a * c);

if sqroot > 0
	if b > 0
		sinU = (-b + sqroot ) / (2 * a);
		dsinUdt = (-dbdt + 1/2 * 1/sqroot * (2*b*dbdt -4*a*dcdt) ) / (2 * a);
		d2sinUdt2 = (-d2bdt2 - 1/4 * 1/sqroot^3 * (2*b*dbdt -4*a*dcdt)^2 + 1/2 * 1/sqroot * (2*dbdt^2 + 2*b*d2bdt2 -4*a*d2cdt2) ) / (2 * a); 
	else
		sinU = (-b - sqroot ) / (2 * a);
		dsinUdt = (-dbdt - 1/2 * 1/sqroot * (2*b*dbdt -4*a*dcdt) ) / (2 * a);
		d2sinUdt2 = (-d2bdt2 + 1/4 * 1/sqroot^3 * (2*b*dbdt -4*a*dcdt)^2 - 1/2 * 1/sqroot * (2*dbdt^2 + 2*b*d2bdt2 -4*a*d2cdt2) ) / (2 * a); 
	end
else
	sinU = -b / (2 * a);
	dsinUdt = -dbdt / (2 * a);
	d2sinUdt2 = -d2bdt2 / (2 * a); 
end	

if sinU > 1
	sinU = 1;
elseif sinU < -1
	sinU = -1;
end

U = asin(sinU);

theta1_5_corr = 2 * U;
vel1_5_corr = 2 / sqrt(1 - sinU^2) * dsinUdt;
acc1_5_corr = 2 / (1 - sinU^2)^(3/2) * sinU * (dsinUdt)^2 + 2 / sqrt(1 - sinU^2) * d2sinUdt2;

angle_corr = - theta1_5_corr;
vel_corr = - vel1_5_corr;
acc_corr = - acc1_5_corr;

== matlab function Bruening_4t_showshuffle/DataLogging/Poll KINARM/createKINData/bitpack ==
  data: statusInts output; statuses input
function statusInts = fcn(statuses)
    statusInts = [0, statuses(5:end)'];

% STATUS_FUNCTIONING = uint32(0);
% STATUS_READY = uint32(1);
% STATUS_FAULTED = uint32(2);

    motorInt = uint32(0);
    for n=1:4
        motorInt = bitor(motorInt, bitshift(statuses(n), (n-1)*2));
    end
    statusInts(1) = uint32(motorInt);
end

== matlab function Bruening_4t_showshuffle/DataLogging/Poll KINARM/createKINData/record errors ==
  data: newMessage output; ECATMessages input; cycle input; step_time input; sentMessageCount output
function [newMessage, sentMessageCount] = fcn(ECATMessages, cycle, step_time)

    persistent lastECATMessages outCount memoryBuffer waitingMsgCount sentCount
    
    if isempty(lastECATMessages)
        lastECATMessages = ECATMessages;
        memoryBuffer = zeros(50, 6);
        waitingMsgCount = 0;
        outCount = 0;
        sentCount = 0;
    end
    
    stepsPerFrame = 0.001 / step_time;

    %copy over the errors from ethercat drives
    for drive=1:4
        if waitingMsgCount >= 50
            continue;
        end
        
        if ECATMessages(drive, 3) ~= lastECATMessages(drive, 3) && ECATMessages(drive, 3) ~= 0
            waitingMsgCount = waitingMsgCount + 1;
            memoryBuffer(waitingMsgCount,:) = [cycle, ECATMessages(drive,1), ECATMessages(drive,2), ECATMessages(drive,3), ECATMessages(drive, 4), ECATMessages(drive,5)];
        end
    end
    
    newMessage = zeros(1,6);
    %if we have an error to send we must send it for a few frames because we only send
    %some frames to the GUI computer. The only safe way to handle this is to count
    %the number of real-time frames vs the frequency we send to the GUI computer on.
    %I wanted to use the actual frame number we send to the GUI, but the trouble is
    %we don't know which of the kinematic frames gets sent to the GUI, it's just one
    %of the 2 or 4 that happens for each frame we send to the GUI. 
    %So instead here I cop out and just count 2 or 4 frames and then send something new.
    if waitingMsgCount > 0
        newMessage = memoryBuffer(1,:);
        outCount = outCount + 1;
        
        %we've sent the frame enough times...
        if outCount >= stepsPerFrame
            %shift the list so the first row is the next thing to send.
            memoryBuffer(1:end-1,:) = memoryBuffer(2:end,:);
            waitingMsgCount = waitingMsgCount - 1;
            sentCount = sentCount + 1;
            outCount = 0;  
            
            %if we still have another frame to send then copy it out..
            if waitingMsgCount > 0
                newMessage = memoryBuffer(1,:);
                outCount = 1;
            end
        end
    end
    
    lastECATMessages = ECATMessages;
    sentMessageCount = sentCount;
end
